simulink model "Infinion"  (R2021a)
settings: Solver=FixedStepAuto  StartTime=0.0  StopTime=3  FixedStep=0.02  RelTol=1e-3
undefined symbols (not defined in the file): aero, Earth, WGS84
libraries: aerolibconvert2 x5, aerolibasang x3, aerolibadyn x2, shared6dof x1, aerolibtransform2 x1
settings Model: Creator=fberbari  LastModifiedBy=nixon
settings SolverCC: AlgebraicLoopSolver=TrustRegion
settings DataIOCC: ReturnWorkspaceOutputs=off
settings OptimizationCC: ZeroExternalMemoryAtStartup=off  ZeroInternalMemoryAtStartup=off
settings DebuggingCC: SFMachineParentedDataDiag=warning  ArithmeticOperatorsInVariantConditions=warning
settings SFSimCC: DefaultCustomCodeFunctionArrayLayout=Row-major  CustomCodeUndefinedFunction=UseInterfaceOnly  SimTargetLang=C++
settings RTWCC: GenCodeOnly=on  PackageGeneratedCodeAndArtifacts=on  PackageName=GeneratedCCode.zip  Toolchain=MinGW64 | gmake (64-bit Windows)  TargetLang=C++
settings GRTTargetCC: TargetLangStandard=C++03 (ISO)  MatFileLogging=off  CodeInterfacePackaging=C++ class

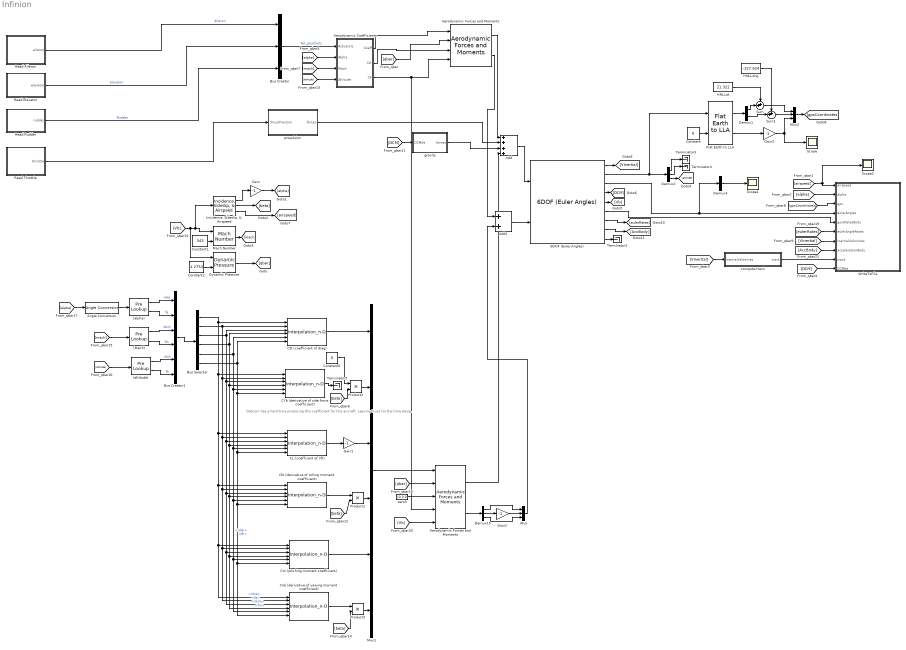
== system Infinion ==
  note: Datcom has a hard time producing this coefficient for this aircraft. Leaving it out for the time being.
  (Mach) : PreLookup  BreakpointsData=aero{1}.mach  BeginIndexSearchUsingPreviousIndexResult=on  ExtrapMethod=Linear  DiagnosticForOutOfRangeInput=Warning  IndexDataTypeStr=int32  FractionDataTypeStr=double
  (alpha) : PreLookup  BreakpointsData=aero{1}.alpha  BeginIndexSearchUsingPreviousIndexResult=on  ExtrapMethod=Linear  DiagnosticForOutOfRangeInput=Warning  IndexDataTypeStr=int32  FractionDataTypeStr=double
  (altitude) : PreLookup  BreakpointsData=aero{1}.alt  BeginIndexSearchUsingPreviousIndexResult=on  ExtrapMethod=Linear  DiagnosticForOutOfRangeInput=Warning  IndexDataTypeStr=int32  FractionDataTypeStr=double
  6DOF (Euler Angles) : shared6dof/6DOF (Euler Angles)  units=Metric (MKS)  mtype=Fixed  rep=Euler Angles  xme_0=[0 0 1000]  Vm_0=[30 0 0]  eul_0=[0 0 0]  pm_0=[0 0 0]  mass_0=1.9  mass_e=0.5  mass_f=2.0  inertia=[0.33 0 0; 0 0.4 0; 0 0 0.66]  inertia_e=eye(3)  inertia_f=2*eye(3)  k_quat=1.0  vre_flag=on  abi_flag=on  aMode=0  xme_statename=''  Vm_statename=''  eul_statename=''  quat_statename=''  pm_statename=''  mass_statename=''
      settings: SourceProductBaseCode=AE,PW,DR,MT,UV,VE
  Add : Sum  Inputs=++++
  Add1 : Sum
  Aerodynamic Coefficients : Subsystem
  Aerodynamic Forces and Moments : aerolibadyn/Aerodynamic Forces and Moments   inputAxes=Wind  outputForceAxes=Body  outputMomentAxes=Body  S=aero{1}.sref  b=aero{1}.blref  cbar=aero{1}.cbar
  "Aerodynamic Forces and Moments " : aerolibadyn/Aerodynamic Forces and Moments   inputAxes=Body  outputForceAxes=Body  outputMomentAxes=Body  S=aero{1}.sref  b=aero{1}.blref  cbar=aero{1}.cbar
  Angle Conversion : aerolibconvert2/Angle Conversion  IU=rad  OU=deg
  Bus Creator : BusCreator  Inputs=3
  Bus Creator1 : BusCreator  Inputs=6
  Bus Selector : BusSelector  OutputSignals=idxa,fa,idxm,fm,idxh,fh
  CD (coefficient of drag) : Interpolation_n-D  NumberOfTableDimensions=3  Table="permute(aero{1}.cd,[1  2  3])"  DiagnosticForOutOfRangeInput=Warning  OutDataTypeStr=double
      settings: InputPortMap=u0,u1,u2,u3,u4,u5
  CL (coeffcient of lift) : Interpolation_n-D  NumberOfTableDimensions=3  Table="permute(aero{1}.cl,[1  2  3])"  DiagnosticForOutOfRangeInput=Warning  OutDataTypeStr=double
      settings: InputPortMap=u0,u1,u2,u3,u4,u5
  CYb (derivative of side force coefficient) : Interpolation_n-D  NumberOfTableDimensions=3  Table="permute(aero{1}.cyb,[1  2  3])"  DiagnosticForOutOfRangeInput=Warning  OutDataTypeStr=double
      settings: InputPortMap=u0,u1,u2,u3,u4,u5
  Clb (derivative of rolling moment coefficient) : Interpolation_n-D  NumberOfTableDimensions=3  Table="permute(aero{1}.clb,[1  2  3])"  DiagnosticForOutOfRangeInput=Warning  OutDataTypeStr=double
      settings: InputPortMap=u0,u1,u2,u3,u4,u5
  Cm (pitching moment coefficient) : Interpolation_n-D  NumberOfTableDimensions=3  Table="permute(aero{1}.cm,[1  2  3])"  DiagnosticForOutOfRangeInput=Warning  OutDataTypeStr=double
      settings: InputPortMap=u0,u1,u2,u3,u4,u5
  Cnb (derivative of yawing moment coefficient) : Interpolation_n-D  NumberOfTableDimensions=3  Table="permute(aero{1}.cnb,[1  2  3])"  DiagnosticForOutOfRangeInput=Warning  OutDataTypeStr=double
      settings: InputPortMap=u0,u1,u2,u3,u4,u5
  Constant : Constant  Value=0
  Constant1 : Constant  Value=343
  Constant2 : Constant  Value=1.2754
  Constant5 : Constant  Value=0
  Demux1 : Demux  Outputs=2
  Demux15 : Demux  Outputs=3
  Demux2 : Demux  Outputs=3
  Demux3 : Demux  Outputs=3
  Dynamic Pressure : aerolibasang/Dynamic Pressure
  Flat Earth to LLA : aerolibtransform2/Flat Earth to LLA  units=Metric (MKS)  ptype=Earth (WGS84)  F=1/298.257223563  R=6378137  refPosPort=off  LL0=[0 0]  psi=0
  Gain{,1..3} (4 alike) : Gain  Gain=-1
  HNLLat : Constant  Value=21.322
  HNLLong : Constant  Value=-157.924
  "Incidence, Sideslip, & Airspeed" : aerolibasang/Incidence, Sideslip, & Airspeed
  Mach Number : aerolibasang/Mach Number
      settings: SourceProductBaseCode=AE
  Mux : Mux  Inputs=3
  Mux1 : Mux  Inputs=6
  Mux2 : Mux  Inputs=3
  Product1 : Product  RndMeth=Zero
  Product2 : Product  RndMeth=Zero
  Product3 : Product  RndMeth=Zero
  Read Aileron : MATLAB Function  TreatAsAtomicUnit=on
  Read Elevator : MATLAB Function  TreatAsAtomicUnit=on
  Read Rudder : MATLAB Function  TreatAsAtomicUnit=on
  Read Throttle : MATLAB Function  TreatAsAtomicUnit=on
  Scope : Scope
  Scope1 : Scope
  Scope2 : Scope
  Sum : Sum  Inputs=++|
  Sum1 : Sum  Inputs=++|
  Terminator{2..5} (4 alike) : Terminator
  WriteToFile : MATLAB Function  TreatAsAtomicUnit=on
  compute track : MATLAB Function  TreatAsAtomicUnit=on
  gravity : MATLAB Function  TreatAsAtomicUnit=on
  propulsion : MATLAB Function  TreatAsAtomicUnit=on
  zero3 : Constant  Value=[0 0 0]
  wires:
  Mux/1 -> Add1/2
  Gain2/1 -> Mux/2
  Demux15/1 -> Mux/1
  Demux15/3 -> Mux/3
  Gain1/1 -> Mux1/3
  Demux15/2 -> Gain2/1
  [beta] -> Product1/2
  [Vb] -> Aerodynamic Forces and Moments/5
  Angle Conversion/1 -> (alpha)/1
  "Incidence, Sideslip, & Airspeed"/1 -> Gain/1
  [qbar] -> Aerodynamic Forces and Moments/2
  Bus Selector/6 -> Cnb (derivative of yawing moment coefficient)/6, Cm (pitching moment coefficient)/6, Clb (derivative of rolling moment coefficient)/6, CL (coeffcient of lift)/6, CYb (derivative of side force coefficient)/6, CD (coefficient of drag)/6  "<fh>"
  zero3/1 -> Aerodynamic Forces and Moments/3
  Bus Selector/5 -> CD (coefficient of drag)/5, Cnb (derivative of yawing moment coefficient)/5, Cm (pitching moment coefficient)/5, Clb (derivative of rolling moment coefficient)/5, CL (coeffcient of lift)/5, CYb (derivative of side force coefficient)/5  "<idxh>"
  Cm (pitching moment coefficient)/1 -> Mux1/5
  Product3/1 -> Mux1/6
  Product1/1 -> Mux1/4
  Cnb (derivative of yawing moment coefficient)/1 -> Product3/1
  Product2/1 -> Mux1/2
  Bus Selector/1 -> CD (coefficient of drag)/1, CYb (derivative of side force coefficient)/1, Clb (derivative of rolling moment coefficient)/1, Cnb (derivative of yawing moment coefficient)/1, Cm (pitching moment coefficient)/1, CL (coeffcient of lift)/1  "<idxa>"
  Bus Selector/2 -> CD (coefficient of drag)/2, Cnb (derivative of yawing moment coefficient)/2, Cm (pitching moment coefficient)/2, Clb (derivative of rolling moment coefficient)/2, CL (coeffcient of lift)/2, CYb (derivative of side force coefficient)/2  "<fa>"
  CL (coeffcient of lift)/1 -> Gain1/1
  Read Elevator/1(elevator) -> Bus Creator/2  "Elevator"
  gravity/1(forces) -> Add/3
  Bus Selector/3 -> CD (coefficient of drag)/3, Cnb (derivative of yawing moment coefficient)/3, Cm (pitching moment coefficient)/3, Clb (derivative of rolling moment coefficient)/3, CL (coeffcient of lift)/3, CYb (derivative of side force coefficient)/3  "<idxm>"
  CD (coefficient of drag)/1 -> Mux1/1
  Bus Selector/4 -> CD (coefficient of drag)/4, Cnb (derivative of yawing moment coefficient)/4, Cm (pitching moment coefficient)/4, Clb (derivative of rolling moment coefficient)/4, CL (coeffcient of lift)/4, CYb (derivative of side force coefficient)/4  "<fm>"
  Read Aileron/1(aileron) -> Bus Creator/1  "Aileron"
  Constant2/1 -> Dynamic Pressure/2
  [DCM] -> gravity/1(DCMbe)
  6DOF (Euler Angles)/5 -> [Vb]
  Bus Creator/1 -> Aerodynamic Coefficients/1(Actuators)  "Act_positions"
  Dynamic Pressure/1 -> [qbar]
  6DOF (Euler Angles)/2 -> Flat Earth to LLA/1, Demux2/1
  "Incidence, Sideslip, & Airspeed"/2 -> [beta]
  [qbar] -> "Aerodynamic Forces and Moments "/2
  Aerodynamic Coefficients/2(CG) -> "Aerodynamic Forces and Moments "/3
  Mach Number/1 -> [mach]
  [Vb] -> Dynamic Pressure/1, "Incidence, Sideslip, & Airspeed"/1, Mach Number/1
  Clb (derivative of rolling moment coefficient)/1 -> Product1/1
  [beta] -> Product3/2
  Aerodynamic Coefficients/3(CP) -> Aerodynamic Forces and Moments/4, "Aerodynamic Forces and Moments "/4
  Aerodynamic Coefficients/1(Coeff) -> "Aerodynamic Forces and Moments "/1
  Read Rudder/1(rudder) -> Bus Creator/3  "Rudder"
  Gain/1 -> [alpha]
  [alpha] -> Angle Conversion/1
  (alpha)/1 -> Bus Creator1/1  "idxa"
  Constant1/1 -> Mach Number/2
  (Mach)/1 -> Bus Creator1/3  "idxm"
  Demux2/3 -> [altitude]
  Mux1/1 -> Aerodynamic Forces and Moments/1
  [altitude] -> Aerodynamic Coefficients/4(Altitude)
  [mach] -> Aerodynamic Coefficients/3(Mach)
  [mach] -> (Mach)/1
  (altitude)/1 -> Bus Creator1/5  "idxh"
  Aerodynamic Forces and Moments/2 -> Demux15/1
  [altitude] -> (altitude)/1
  propulsion/1(forces) -> Add/2
  (altitude)/2 -> Bus Creator1/6  "fh"
  Aerodynamic Forces and Moments/1 -> Add/4
  [alpha] -> Aerodynamic Coefficients/2(Alpha)
  6DOF (Euler Angles)/4 -> [DCM]
  (alpha)/2 -> Bus Creator1/2  "fa"
  [beta] -> Product2/2
  Bus Creator1/1 -> Bus Selector/1
  (Mach)/2 -> Bus Creator1/4  "fm"
  "Incidence, Sideslip, & Airspeed"/3 -> [airspeed]
  [airspeed] -> Scope2/1, WriteToFile/1(airspeed)
  [alpha] -> WriteToFile/2(alpha)
  6DOF (Euler Angles)/3 -> Demux3/1, WriteToFile/4(eulerAngles)
  6DOF (Euler Angles)/6 -> WriteToFile/5(gyroRatesBody)
  [DCM] -> WriteToFile/10(DCMbe)
  6DOF (Euler Angles)/9 -> Terminator2/1
  Demux2/2 -> Terminator4/1
  Demux2/1 -> Terminator3/1
  Read Throttle/1(throttle) -> propulsion/1(thrustFraction)
  Flat Earth to LLA/1 -> Demux1/1
  Mux2/1 -> [gpsCoordinates]
  Constant/1 -> Flat Earth to LLA/2
  [gpsCoordinates] -> WriteToFile/3(gps)
  Demux1/1 -> Sum/2
  Demux1/2 -> Sum1/2
  Sum1/1 -> Mux2/2
  Sum/1 -> Mux2/1
  HNLLat/1 -> Sum/1
  HNLLong/1 -> Sum1/1
  Flat Earth to LLA/2 -> Gain3/1
  Gain3/1 -> Mux2/3, Scope/1
  Constant5/1 -> Product2/1
  CYb (derivative of side force coefficient)/1 -> Terminator5/1
  "Aerodynamic Forces and Moments "/2 -> Add1/1
  "Aerodynamic Forces and Moments "/1 -> Add/1
  Demux3/2 -> Scope1/1
  [VInertial] -> compute track/1(inertialVelocities)
  [VInertial] -> WriteToFile/7(inertialVelocities)
  6DOF (Euler Angles)/7 -> [eulerRates]
  [eulerRates] -> WriteToFile/6(eulerAngleRates)
  6DOF (Euler Angles)/8 -> [AccBody]
  [AccBody] -> WriteToFile/8(accelerationBody)
  compute track/1(track) -> WriteToFile/9(track)
  6DOF (Euler Angles)/1 -> [VInertial]
  Add/1 -> 6DOF (Euler Angles)/1
  Add1/1 -> 6DOF (Euler Angles)/2

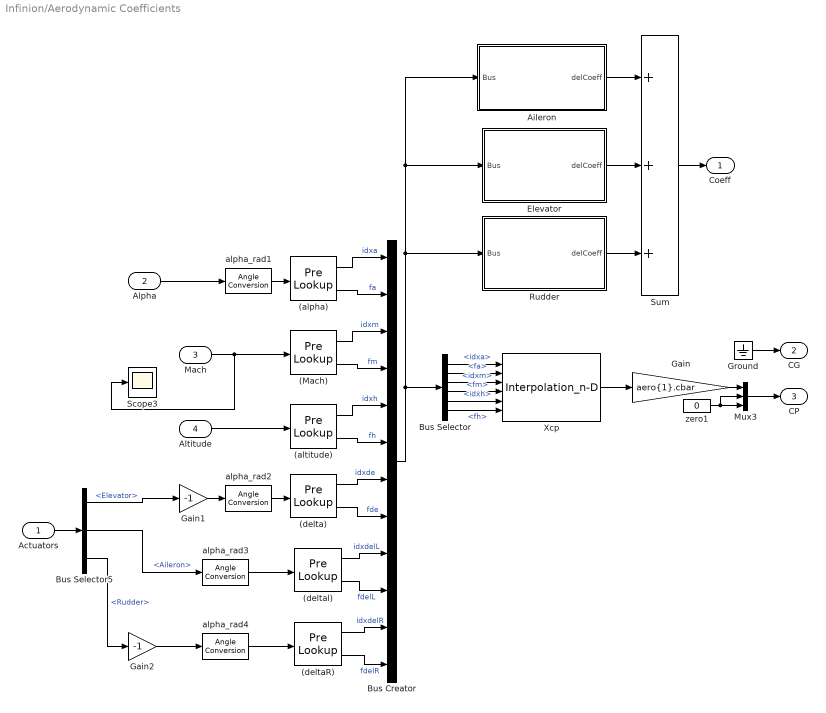
== system Infinion/Aerodynamic Coefficients ==
  Actuators : Inport
  Alpha : Inport  Port=2
  Mach : Inport  Port=3
  Altitude : Inport  Port=4
  (Mach) : PreLookup  BreakpointsData=aero{1}.mach  BeginIndexSearchUsingPreviousIndexResult=on  ExtrapMethod=Linear  IndexDataTypeStr=int32  FractionDataTypeStr=double
  (alpha) : PreLookup  BreakpointsData=aero{1}.alpha  BeginIndexSearchUsingPreviousIndexResult=on  ExtrapMethod=Linear  IndexDataTypeStr=int32  FractionDataTypeStr=double
  (altitude) : PreLookup  BreakpointsData=aero{1}.alt  BeginIndexSearchUsingPreviousIndexResult=on  ExtrapMethod=Linear  IndexDataTypeStr=int32  FractionDataTypeStr=double
  (delta) : PreLookup  BreakpointsData=aero{1}.delta  BeginIndexSearchUsingPreviousIndexResult=on  ExtrapMethod=Linear  IndexDataTypeStr=int32  FractionDataTypeStr=double
  (deltaR) : PreLookup  BreakpointsData=aero{3}.delta  BeginIndexSearchUsingPreviousIndexResult=on  ExtrapMethod=Linear  IndexDataTypeStr=int32  FractionDataTypeStr=double
  (deltal) : PreLookup  BreakpointsData=aero{2}.deltal  BeginIndexSearchUsingPreviousIndexResult=on  ExtrapMethod=Linear  IndexDataTypeStr=int32  FractionDataTypeStr=double
  Aileron : Subsystem
  Bus Creator : BusCreator  Inputs=12
  Bus Selector : BusSelector  OutputSignals=idxa,fa,idxm,fm,idxh,fh
  Bus Selector5 : BusSelector  OutputSignals=Elevator,Aileron,Rudder
  Elevator : Subsystem
  Gain : Gain  Gain=aero{1}.cbar
  Gain1 : Gain  Gain=-1
  Gain2 : Gain  Gain=-1
  Ground : Ground
  Mux3 : Mux  Inputs=3
  Rudder : Subsystem
  Scope3 : Scope
  Sum : Sum  Inputs=3  InputSameDT=on  SaturateOnIntegerOverflow=on  OutDataTypeStr=Inherit: Same as first input
  Xcp : Interpolation_n-D  NumberOfTableDimensions=3  Table="permute(aero{1}.xcp,[1  2  3])"  OutDataTypeStr=double
      settings: InputPortMap=u0,u1,u2,u3,u4,u5
  alpha_rad{1..4} (4 alike) : aerolibconvert2/Angle Conversion  IU=rad  OU=deg
  zero1 : Constant  Value=0
  Coeff : Outport  InitialOutput=0  VectorParamsAs1DForOutWhenUnconnected=off
  CG : Outport  Port=2  PortDimensions=3  InitialOutput=0  VectorParamsAs1DForOutWhenUnconnected=off
  CP : Outport  Port=3  PortDimensions=3  InitialOutput=0  VectorParamsAs1DForOutWhenUnconnected=off
  wires:
  Sum/1 -> Coeff/1
  Actuators/1 -> Bus Selector5/1
  Ground/1 -> CG/1
  Mux3/1 -> CP/1
  Xcp/1 -> Gain/1
  zero1/1 -> Mux3/2, Mux3/3
  Gain/1 -> Mux3/1
  (alpha)/2 -> Bus Creator/2  "fa"
  (Mach)/2 -> Bus Creator/4  "fm"
  (altitude)/2 -> Bus Creator/6  "fh"
  (altitude)/1 -> Bus Creator/5  "idxh"
  (Mach)/1 -> Bus Creator/3  "idxm"
  (alpha)/1 -> Bus Creator/1  "idxa"
  Bus Selector/1 -> Xcp/1  "<idxa>"
  Bus Selector/2 -> Xcp/2  "<fa>"
  Bus Selector/3 -> Xcp/3  "<idxm>"
  Bus Selector/4 -> Xcp/4  "<fm>"
  Bus Selector/5 -> Xcp/5  "<idxh>"
  Bus Selector/6 -> Xcp/6  "<fh>"
  Bus Creator/1 -> Bus Selector/1, Rudder/1(Bus), Elevator/1(Bus), Aileron/1(Bus)
  Mach/1 -> Scope3/1, (Mach)/1
  Altitude/1 -> (altitude)/1
  alpha_rad1/1 -> (alpha)/1
  Aileron/1(delCoeff) -> Sum/1
  Elevator/1(delCoeff) -> Sum/2
  Rudder/1(delCoeff) -> Sum/3
  (delta)/1 -> Bus Creator/7  "idxde"
  (delta)/2 -> Bus Creator/8  "fde"
  alpha_rad2/1 -> (delta)/1
  Gain1/1 -> alpha_rad2/1
  Bus Selector5/1 -> Gain1/1  "<Elevator>"
  (deltal)/1 -> Bus Creator/9  "idxdelL"
  (deltal)/2 -> Bus Creator/10  "fdelL"
  alpha_rad3/1 -> (deltal)/1
  Bus Selector5/2 -> alpha_rad3/1  "<Aileron>"
  Alpha/1 -> alpha_rad1/1
  alpha_rad4/1 -> (deltaR)/1
  (deltaR)/1 -> Bus Creator/11  "idxdelR"
  (deltaR)/2 -> Bus Creator/12  "fdelR"
  Gain2/1 -> alpha_rad4/1
  Bus Selector5/3 -> Gain2/1  "<Rudder>"

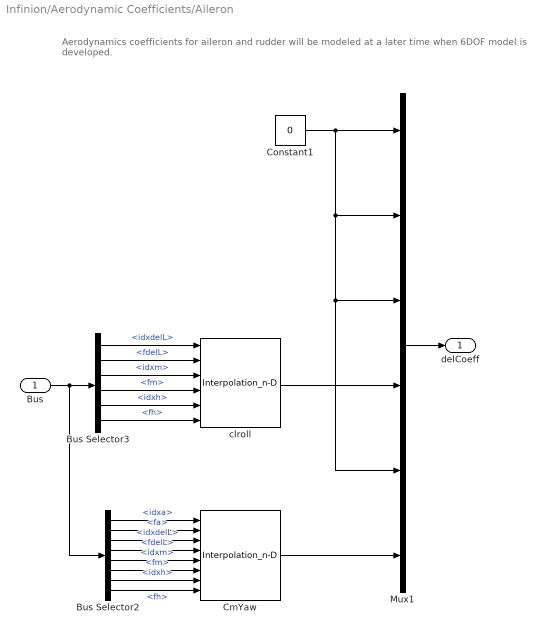
== system Infinion/Aerodynamic Coefficients/Aileron ==
  note: Aerodynamics coefficients for aileron and rudder will be modeled at a later time when 6DOF model is developed.
  Bus : Inport
  Bus Selector2 : BusSelector  OutputSignals=idxa,fa,idxdelL,fdelL,idxm,fm,idxh,fh
  Bus Selector3 : BusSelector  OutputSignals=idxdelL,fdelL,idxm,fm,idxh,fh
  "CmYaw " : Interpolation_n-D  NumberOfTableDimensions=4  Table=aero{2}.cn_asy  RemoveProtectionIndex=on
      settings: InputPortMap=u0,u1,u2,u3,u4,u5,u6,u7
  Constant1 : Constant  Value=0
  Mux1 : Mux  Inputs=6
  clroll : Interpolation_n-D  NumberOfTableDimensions=3  Table="permute(aero{2}.clroll,[1  2  3])"  RemoveProtectionIndex=on
      settings: InputPortMap=u0,u1,u2,u3,u4,u5
  delCoeff : Outport  VectorParamsAs1DForOutWhenUnconnected=off
  wires:
  Mux1/1 -> delCoeff/1
  Constant1/1 -> Mux1/1, Mux1/2, Mux1/3, Mux1/5
  clroll/1 -> Mux1/4
  Bus/1 -> Bus Selector2/1, Bus Selector3/1
  Bus Selector3/1 -> clroll/1  "<idxdelL>"
  Bus Selector3/2 -> clroll/2  "<fdelL>"
  Bus Selector3/3 -> clroll/3  "<idxm>"
  Bus Selector3/4 -> clroll/4  "<fm>"
  Bus Selector3/5 -> clroll/5  "<idxh>"
  Bus Selector3/6 -> clroll/6  "<fh>"
  "CmYaw "/1 -> Mux1/6
  Bus Selector2/1 -> "CmYaw "/1  "<idxa>"
  Bus Selector2/2 -> "CmYaw "/2  "<fa>"
  Bus Selector2/3 -> "CmYaw "/3  "<idxdelL>"
  Bus Selector2/4 -> "CmYaw "/4  "<fdelL>"
  Bus Selector2/5 -> "CmYaw "/5  "<idxm>"
  Bus Selector2/6 -> "CmYaw "/6  "<fm>"
  Bus Selector2/7 -> "CmYaw "/7  "<idxh>"
  Bus Selector2/8 -> "CmYaw "/8  "<fh>"

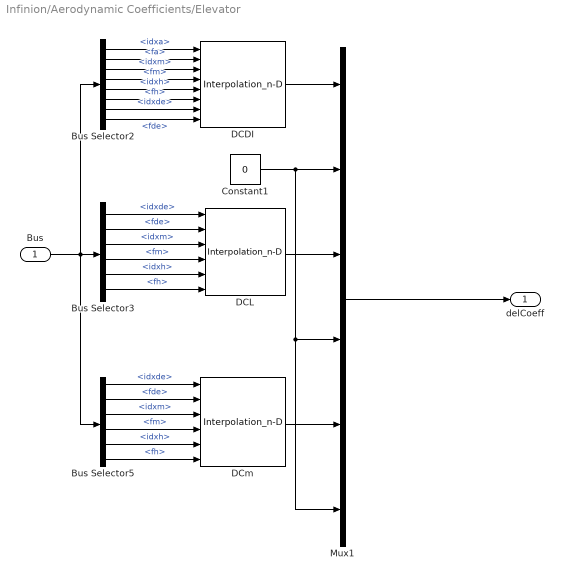
== system Infinion/Aerodynamic Coefficients/Elevator ==
  Bus : Inport
  Bus Selector2 : BusSelector  OutputSignals=idxa,fa,idxm,fm,idxh,fh,idxde,fde
  Bus Selector3 : BusSelector  OutputSignals=idxde,fde,idxm,fm,idxh,fh
  Bus Selector5 : BusSelector  OutputSignals=idxde,fde,idxm,fm,idxh,fh
  Constant1 : Constant  Value=0
  DCDI : Interpolation_n-D  NumberOfTableDimensions=4  Table=permute(aero{1}.dcdi_sym,[1 3 4 2 ])  RemoveProtectionIndex=on
      settings: InputPortMap=u0,u1,u2,u3,u4,u5,u6,u7
  DCL : Interpolation_n-D  NumberOfTableDimensions=3  Table="permute(aero{1}.dcl_sym,[1  2  3])"  RemoveProtectionIndex=on
      settings: InputPortMap=u0,u1,u2,u3,u4,u5
  DCm : Interpolation_n-D  NumberOfTableDimensions=3  Table="permute(aero{1}.dcm_sym,[1  2  3])"  RemoveProtectionIndex=on
      settings: InputPortMap=u0,u1,u2,u3,u4,u5
  Mux1 : Mux  Inputs=6
  delCoeff : Outport  VectorParamsAs1DForOutWhenUnconnected=off
  wires:
  Mux1/1 -> delCoeff/1
  Bus/1 -> Bus Selector2/1, Bus Selector3/1, Bus Selector5/1
  DCDI/1 -> Mux1/1
  DCL/1 -> Mux1/3
  DCm/1 -> Mux1/5
  Constant1/1 -> Mux1/2, Mux1/4, Mux1/6
  Bus Selector2/1 -> DCDI/1  "<idxa>"
  Bus Selector2/2 -> DCDI/2  "<fa>"
  Bus Selector3/1 -> DCL/1  "<idxde>"
  Bus Selector3/2 -> DCL/2  "<fde>"
  Bus Selector5/1 -> DCm/1  "<idxde>"
  Bus Selector5/2 -> DCm/2  "<fde>"
  Bus Selector2/3 -> DCDI/3  "<idxm>"
  Bus Selector2/4 -> DCDI/4  "<fm>"
  Bus Selector2/5 -> DCDI/5  "<idxh>"
  Bus Selector2/6 -> DCDI/6  "<fh>"
  Bus Selector2/7 -> DCDI/7  "<idxde>"
  Bus Selector2/8 -> DCDI/8  "<fde>"
  Bus Selector3/3 -> DCL/3  "<idxm>"
  Bus Selector3/4 -> DCL/4  "<fm>"
  Bus Selector3/5 -> DCL/5  "<idxh>"
  Bus Selector3/6 -> DCL/6  "<fh>"
  Bus Selector5/3 -> DCm/3  "<idxm>"
  Bus Selector5/4 -> DCm/4  "<fm>"
  Bus Selector5/5 -> DCm/5  "<idxh>"
  Bus Selector5/6 -> DCm/6  "<fh>"

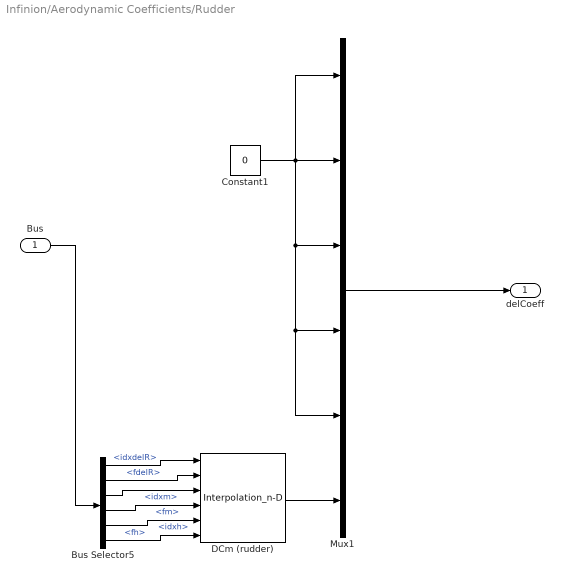
== system Infinion/Aerodynamic Coefficients/Rudder ==
  Bus : Inport
  Bus Selector5 : BusSelector  OutputSignals=idxdelR,fdelR,idxm,fm,idxh,fh
  Constant1 : Constant  Value=0
  DCm (rudder) : Interpolation_n-D  NumberOfTableDimensions=3  Table="permute(aero{3}.dcm_sym,[1  2  3])"  RemoveProtectionIndex=on
      settings: InputPortMap=u0,u1,u2,u3,u4,u5
  Mux1 : Mux  Inputs=6
  delCoeff : Outport  VectorParamsAs1DForOutWhenUnconnected=off
  wires:
  Mux1/1 -> delCoeff/1
  Bus/1 -> Bus Selector5/1
  Bus Selector5/3 -> DCm (rudder)/3  "<idxm>"
  Bus Selector5/4 -> DCm (rudder)/4  "<fm>"
  Bus Selector5/5 -> DCm (rudder)/5  "<idxh>"
  Bus Selector5/6 -> DCm (rudder)/6  "<fh>"
  Constant1/1 -> Mux1/1, Mux1/2, Mux1/3, Mux1/5, Mux1/4
  Bus Selector5/1 -> DCm (rudder)/1  "<idxdelR>"
  Bus Selector5/2 -> DCm (rudder)/2  "<fdelR>"
  DCm (rudder)/1 -> Mux1/6

== matlab function Infinion/WriteToFile ==
  data: airspeed input; alpha input; gps input; eulerAngles input; gyroRatesBody input; eulerAngleRates input; inertialVelocities input; accelerationBody input; track input; DCMbe input
%#codegen
function fcn(airspeed, alpha, gps, eulerAngles, gyroRatesBody, eulerAngleRates, inertialVelocities, accelerationBody, track, DCMbe)

gravityInertial = [0;0;-9.8];
gravityBody = DCMbe * gravityInertial;

airSpeedFile = fopen( 'SensorOutputs/airspeed.txt', 'a' );

aoaFile = fopen( 'SensorOutputs/angleOfAttack.txt', 'a' );

trackFile = fopen( 'SensorOutputs/track.txt', 'a' );

latSpeedFile = fopen( 'SensorOutputs/latitudeSpeed.txt', 'a' );
longSpeedFile = fopen( 'SensorOutputs/longitudeSpeed.txt', 'a' );
rateOfClimbFile = fopen( 'SensorOutputs/rateOfClimb.txt', 'a' );

latFile = fopen( 'SensorOutputs/latitude.txt', 'a' );
longFile = fopen( 'SensorOutputs/longitude.txt', 'a' );
altitudeFile = fopen( 'SensorOutputs/altitude.txt', 'a' );

rollFile = fopen( 'SensorOutputs/roll.txt', 'a' );
pitchFile = fopen( 'SensorOutputs/pitch.txt', 'a' );
yawFile = fopen( 'SensorOutputs/yaw.txt', 'a' );

rollRateFile = fopen( 'SensorOutputs/rollRate.txt', 'a' );
pitchRateFile = fopen( 'SensorOutputs/pitchRate.txt', 'a' );
yawRateFile = fopen( 'SensorOutputs/yawRate.txt', 'a' );

accXFile = fopen( 'SensorOutputs/accX.txt', 'a' );
accYFile = fopen( 'SensorOutputs/accY.txt', 'a' );
accZFile = fopen( 'SensorOutputs/accZ.txt', 'a' );

gyrXFile = fopen( 'SensorOutputs/gyrX.txt', 'a' );
gyrYFile = fopen( 'SensorOutputs/gyrY.txt', 'a' );
gyrZFile = fopen( 'SensorOutputs/gyrZ.txt', 'a' );

fprintf( airSpeedFile,'%f\n',airspeed);

fprintf( aoaFile,'%f\n',alpha);

fprintf( trackFile,'%f\n',track);

fprintf( latSpeedFile,'%f\n',inertialVelocities(1));
fprintf( longSpeedFile,'%f\n',inertialVelocities(2));
fprintf( rateOfClimbFile,'%f\n',inertialVelocities(3));

fprintf( latFile,'%f\n',gps(1));
fprintf( longFile,'%f\n',gps(2));
fprintf( altitudeFile,'%f\n',gps(3));

fprintf( rollFile,'%f\n',eulerAngles(1));
fprintf( pitchFile,'%f\n',eulerAngles(2));
fprintf( yawFile,'%f\n',eulerAngles(3));

fprintf( rollRateFile,'%f\n',eulerAngleRates(1));
fprintf( pitchRateFile,'%f\n',eulerAngleRates(2));
fprintf( yawRateFile,'%f\n',eulerAngleRates(3));

fprintf( accXFile,'%f\n',gravityBody(1) + accelerationBody(1));
fprintf( accYFile,'%f\n',gravityBody(2) + accelerationBody(2));
fprintf( accZFile,'%f\n',gravityBody(3) + accelerationBody(3));

fprintf( gyrXFile,'%f\n',gyroRatesBody(1));
fprintf( gyrYFile,'%f\n',gyroRatesBody(2));
fprintf( gyrZFile,'%f\n',gyroRatesBody(3));

fclose('all');

== matlab function Infinion/Read Aileron ==
  data: aileron output
%#codegen
function aileron = fcn()

s = readfile('ActuatorCommands/aileron.txt');

latestData = lastStr2double(s);

maxAileronDeflect = 0.2618; % radians

aileron = (latestData * maxAileronDeflect) / 100.0;

== matlab function Infinion/Read Throttle ==
  data: throttle output
%#codegen
function throttle = fcn()

s = readfile('ActuatorCommands/throttle.txt');
latestData = lastStr2double(s);

throttle = (latestData / 100.0);

== matlab function Infinion/Read Rudder ==
  data: rudder output
%#codegen
function rudder = fcn()

s = readfile('ActuatorCommands/rudder.txt');
latestData = lastStr2double(s);

maxRudderDeflect = 0.2618; % radians

rudder = (latestData * maxRudderDeflect) / 100.0;

== matlab function Infinion/Read Elevator ==
  data: elevator output
%#codegen
function elevator = fcn()

s = readfile('ActuatorCommands/elevator.txt');
latestData = lastStr2double(s);

maxElevatorDeflect = 0.2618; % radians

elevator = (latestData * maxElevatorDeflect) / 100.0;

== matlab function Infinion/compute track ==
  data: inertialVelocities input; track output
function track = fcn(inertialVelocities)

% We're using longitudinal velocity as the X input so that 0 degrees lines
% up with north
tempTrack = -atan2(inertialVelocities(2), inertialVelocities(1));

if tempTrack < 0
    tempTrack = tempTrack + (2 * pi);
end

track = tempTrack;

== matlab function Infinion/gravity ==
  data: forces output; DCMbe input
%#codegen
function forces  = fcn(DCMbe)

mass = 1.9; % Kg
gravityInertial = [0;0;-9.8*mass];
gravityBody = DCMbe * gravityInertial;

forces = gravityBody;

== matlab function Infinion/propulsion ==
  data: forces output; thrustFraction input
%#codegen
function forces  = fcn(thrustFraction)

percentToThrustFactor = 0.20; % newtons/percent (estimated, if someone 10 years from now comes accross this comment, first of all Hi, I hape your'e having a nice day :). I also hope the fucking pandemic is nothing but a distant memory. Oh yeah and feel free to get legit thrust data).


forces = [(percentToThrustFactor*thrustFraction*100);0;0];
